simulink library "Feeder1_lib"  (Simulink 8.1)
settings: Solver=ode45  StartTime=0.0  StopTime=10.0  RelTol=1e-3
values from neighbouring files (symbols this model uses):
  DER_REL = xlsread('DER_relay.xlsx')    [relay_settings_init.m]
  Ts = 100E-6    (= 0.0001)    [BANSHEE_init.m]    (also in Ghost_init.m)
undefined symbols (not defined in the file or in its folder): CBID, Left, type, V
libraries: breaker_lib x16, powerlib x11, cables_lib x11, transformer_lib x7, Load_lib x6, ssn_lib x6, NREL_Diesel_Genset_lib x2, rtlab x2, relay_modbus_lib x1, powerlib_meascontrol x1, rtio_generic_modbus x1, Motor_InductionMachine_lib x1
settings Model: Creator=re25624  LastModifiedBy=hptb1

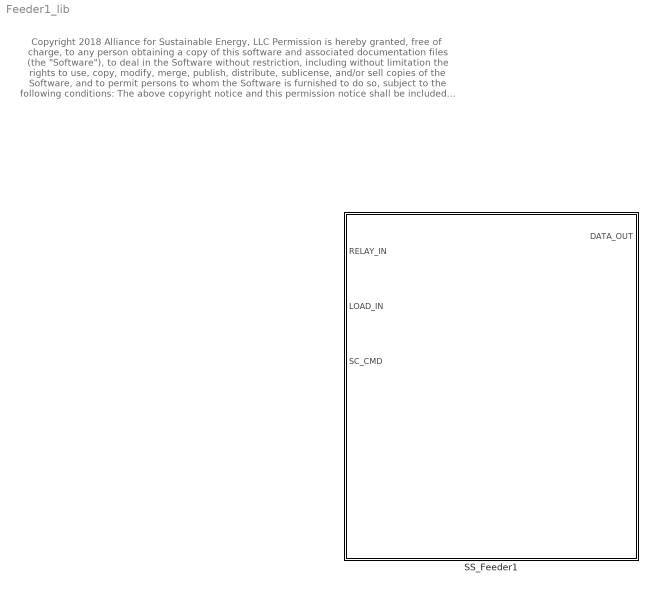
== system Feeder1_lib ==
  note: Copyright 2018 Alliance for Sustainable Energy, LLC
      |
      | Permission is hereby granted, free of charge, to any person obtaining a copy of this software
      | and associated documentation files (the "Software"), to deal in the Software without restriction,
      | including without limitation the rights to use, copy, modify, merge, publish, distribute, sublicense,
      | and/or sell copies of the Software, and to permit persons to whom the Software is furnished to do so,
      | subject to the following conditions:
      |
      | The above copyright notice and this permission notice shall be included in all copies or substantial portions of the Software.
      |
      | THE SOFTWARE IS PROVIDED "AS IS", WITHOUT WARRANTY OF ANY KIND, EXPRESS OR IMPLIED, INCLUDING
      | BUT NOT LIMITED TO THE WARRANTIES OF MERCHANTABILITY, FITNESS FOR A PARTICULAR PURPOSE AND
      | NONINFRINGEMENT. IN NO EVENT SHALL THE AUTHORS, THE COPYRIGHT HOLDERS, THE UNITED STATES,
      | THE UNITED STATES DEPARTMENT OF ENERGY, OR ANY OF THEIR EMPLOYEES BE LIABLE FOR ANY CLAIM,
      | DAMAGES OR OTHER LIABILITY, WHETHER IN AN ACTION OF CONTRACT, TORT OR OTHERWISE, ARISING FROM,
      | OUT OF OR IN CONNECTION WITH THE SOFTWARE OR THE USE OR OTHER DEALINGS IN THE SOFTWARE.
  SS_Feeder1 : Subsystem

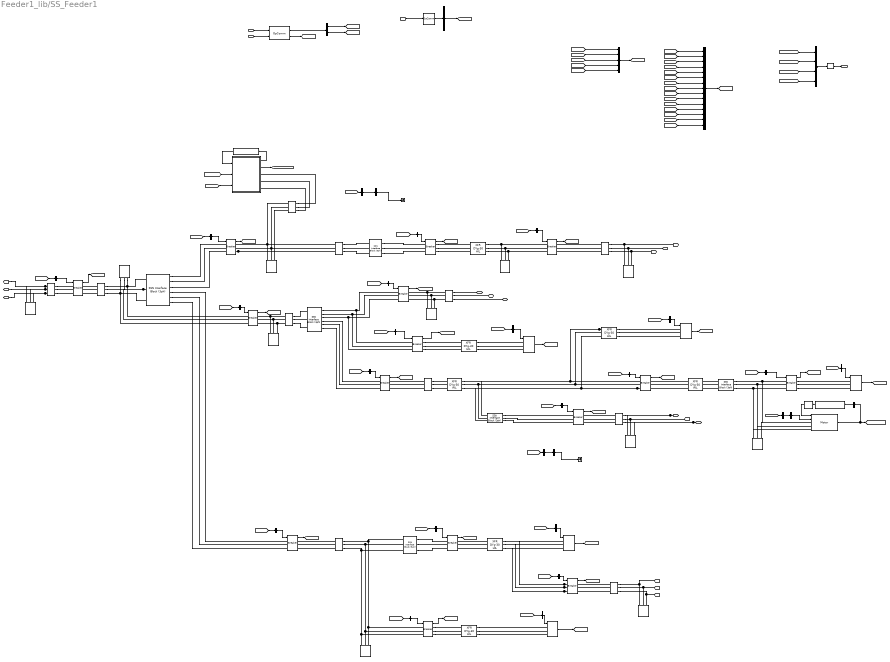
== system Feeder1_lib/SS_Feeder1 ==
  note: Copyright 2018 Alliance for Sustainable Energy, LLC
      |
      | Permission is hereby granted, free of charge, to any person obtaining a copy of this software
      | and associated documentation files (the "Software"), to deal in the Software without restriction,
      | including without limitation the rights to use, copy, modify, merge, publish, distribute, sublicense,
      | and/or sell copies of the Software, and to permit persons to whom the Software is furnished to do so,
      | subject to the following conditions:
      |
      | The above copyright notice and this permission notice shall be included in all copies or substantial portions of the Software.
      |
      | THE SOFTWARE IS PROVIDED "AS IS", WITHOUT WARRANTY OF ANY KIND, EXPRESS OR IMPLIED, INCLUDING
      | BUT NOT LIMITED TO THE WARRANTIES OF MERCHANTABILITY, FITNESS FOR A PARTICULAR PURPOSE AND
      | NONINFRINGEMENT. IN NO EVENT SHALL THE AUTHORS, THE COPYRIGHT HOLDERS, THE UNITED STATES,
      | THE UNITED STATES DEPARTMENT OF ENERGY, OR ANY OF THEIR EMPLOYEES BE LIABLE FOR ANY CLAIM,
      | DAMAGES OR OTHER LIABILITY, WHETHER IN AN ACTION OF CONTRACT, TORT OR OTHERWISE, ARISING FROM,
      | OUT OF OR IN CONNECTION WITH THE SOFTWARE OR THE USE OR OTHER DEALINGS IN THE SOFTWARE.
  note: Copyright 2018 Alliance for Sustainable Energy, LLC
      |
      | Permission is hereby granted, free of charge, to any person obtaining a copy of this software
      | and associated documentation files (the "Software"), to deal in the Software without restriction,
      | including without limitation the rights to use, copy, modify, merge, publish, distribute, sublicense,
      | and/or sell copies of the Software, and to permit persons to whom the Software is furnished to do so,
      | subject to the following conditions:
      |
      | The above copyright notice and this permission notice shall be included in all copies or substantial portions of the Software.
      |
      | THE SOFTWARE IS PROVIDED "AS IS", WITHOUT WARRANTY OF ANY KIND, EXPRESS OR IMPLIED, INCLUDING
      | BUT NOT LIMITED TO THE WARRANTIES OF MERCHANTABILITY, FITNESS FOR A PARTICULAR PURPOSE AND
      | NONINFRINGEMENT. IN NO EVENT SHALL THE AUTHORS, THE COPYRIGHT HOLDERS, THE UNITED STATES,
      | THE UNITED STATES DEPARTMENT OF ENERGY, OR ANY OF THEIR EMPLOYEES BE LIABLE FOR ANY CLAIM,
      | DAMAGES OR OTHER LIABILITY, WHETHER IN AN ACTION OF CONTRACT, TORT OR OTHERWISE, ARISING FROM,
      | OUT OF OR IN CONNECTION WITH THE SOFTWARE OR THE USE OR OTHER DEALINGS IN THE SOFTWARE.
  note: Fault3:
      | Fault Resistance: 0.01Ohm
      | Ground Resistance: 1.73Ohm
      | Snubber resistance: 1E6:
  note: 124kVA to cancel capcitive VARs
      | from stubline
  note: connect to F3
  note: connect to F2
  note: connect to F2
  note: connect to F2
  note: 69kVA to cancel capcitive VARs
      | from stubline
  note: Fault2:
      | Fault Resistance: 0.1Ohm
      | Ground Resistance: 1.73Ohm
      | Snubber resistance: 1E6:
  RELAY_IN : Inport
  LOAD_IN : Inport  Port=2
  SC_CMD : Inport  Port=3
  200 HP chiller compressor : Load_lib/200 HP chiller compressor
  2000 kVA4 : transformer_lib/XFR DYg-30 HIL  Rating=2000  Vp=4160  Vs=480  Z=5.75  XR=5.7
  2000 kVA5 : transformer_lib/XFR DYg-30 HIL  Rating=2000  Vp=4160  Vs=480  Z=5.75  XR=5.7
  2500 kVA : transformer_lib/XFR DYg-30 HIL  Rating=2500  Vp=13800  Vs=480  Z=5.75  XR=6.6
  2500 kVA2 : transformer_lib/XFR DYg-30 HIL  Rating=2500  Vp=13800  Vs=480  Z=5.56  XR=5.52
  3750 kVA1 : transformer_lib/XFR DYg-30 HIL  Rating=3750  Vp=13800  Vs=4160  Z=4.75  XR=11.4
  448 kvar inductor at 13.8kV  to cancel kvar produced by the stublines1 : powerlib/Elements/Three-Phase Parallel RLC Load  LConnTagsString=A|B|C  Configuration=Y (grounded)  NominalVoltage=13800  NominalFrequency=60  ActivePower=10e3  InductivePower=448e3  CapacitivePower=0  Measurements=None  LoadType=constant Z
  5 kvar inductor at 480V  to cancel kvar produced by the stublines : powerlib/Elements/Three-Phase Parallel RLC Load  LConnTagsString=A|B|C  Configuration=Y (grounded)  NominalVoltage=480  NominalFrequency=60  ActivePower=1e3  InductivePower=5e3  CapacitivePower=0  Measurements=None  LoadType=constant Z
  500 kVA2 : transformer_lib/XFR DYg-30 HIL  Rating=500  Vp=13800  Vs=480  Z=5  XR=4.9
  500 kVA3 : transformer_lib/XFR DYg-30 HIL  Rating=500  Vp=13800  Vs=208  Z=5  XR=4.9
  500kcmil-Mutual1 : cables_lib/500kcmil-Mutual  length=1000  par_sets=1  ratio=3
  500kcmil-Mutual9 : cables_lib/500kcmil-Mutual  length=100  par_sets=1  ratio=3
  9 kvar inductor at 480V  to cancel kvar produced by the stublines2 : powerlib/Elements/Three-Phase Parallel RLC Load  LConnTagsString=A|B|C  Configuration=Y (grounded)  NominalVoltage=480  NominalFrequency=60  ActivePower=1e3  InductivePower=9e3  CapacitivePower=0  Measurements=None  LoadType=constant Z
  Bus Creator2 : BusCreator
  Bus Creator3 : BusCreator  Inputs=5
  Bus Creator5 : BusCreator  Inputs=15
  Bus Selector : BusSelector  OutputSignals=motor
  Bus Selector1 : BusSelector  OutputSignals=F1_CB_12
  Bus Selector10 : BusSelector  OutputSignals=F1_CB_2
  Bus Selector11 : BusSelector  OutputSignals=F1_CB_1
  Bus Selector12 : BusSelector  OutputSignals=F1_CB_5
  Bus Selector13 : BusSelector  OutputSignals=F1_CB_3
  Bus Selector14 : BusSelector  OutputSignals=F1_CB_6
  Bus Selector15 : BusSelector  OutputSignals=F1_CB_7
  Bus Selector16 : BusSelector  OutputSignals=F1_CB_10
  Bus Selector17 : BusSelector  OutputSignals=F1_CB_11
  Bus Selector18 : BusSelector  OutputSignals=F1_CB_9
  Bus Selector19 : BusSelector  OutputSignals=F1_CB_14
  Bus Selector2 : BusSelector  OutputSignals=F1_CB_4
  Bus Selector20 : BusSelector  OutputSignals=Gen1
  Bus Selector21 : BusSelector  OutputSignals=LoadProfile,TestSeq
  Bus Selector22 : BusSelector  OutputSignals=RPM
  Bus Selector23 : BusSelector  OutputSignals=ena1
  Bus Selector24 : BusSelector  OutputSignals=fault
  Bus Selector25 : BusSelector  OutputSignals=loc2
  Bus Selector26 : BusSelector  OutputSignals=F1_PCC
  Bus Selector27 : BusSelector  OutputSignals=fault
  Bus Selector28 : BusSelector  OutputSignals=loc3
  Bus Selector3 : BusSelector  OutputSignals=I2
  Bus Selector4 : BusSelector  OutputSignals=C2
  Bus Selector5 : BusSelector  OutputSignals=P1
  Bus Selector6 : BusSelector  OutputSignals=C1
  Bus Selector7 : BusSelector  OutputSignals=I1
  Bus Selector8 : BusSelector  OutputSignals=F1_CB_13
  Bus Selector9 : BusSelector  OutputSignals=F1_CB_8
  C{1..2,108..109} (4 alike) : cables_lib/500kcmil-Mutual  length=10  par_sets=1  ratio=3
  C101 : cables_lib/500kcmil-Mutual  length=1800  par_sets=1  ratio=3
  C102 : cables_lib/500kcmil-Mutual  length=5500  par_sets=1  ratio=3
  C103 : cables_lib/4//0AWG-Mutual  length=1000  par_sets=1  ratio=3
  C104 : cables_lib/500kcmil-Mutual  length=3000  par_sets=1  ratio=3
  C106 : cables_lib/500kcmil-Mutual  length=1500  par_sets=1  ratio=3
  Critical_1 : Load_lib/Dynamic_Load  V=480  kVA=1200  PF=0.9  Ts=Ts
  Critical_2 : Load_lib/Dynamic_Load  V=480  kVA=1500  PF=0.9  Ts=Ts
  Diesel_Generator1 : Subsystem
  F1_CB_{1..14} (14 alike) : breaker_lib/Breaker  Ts=Ts  mech_delay=cb_mech_delay
  F1_PCC : breaker_lib/Breaker  Ts=Ts  mech_delay=cb_mech_delay
  First-Order Filter : powerlib_meascontrol/Filters/First-Order Filter  FilterType=Lowpass  Tc=10e-3  Ts=Ts  Initialize=on  Vac_Init=[0, 0, 60]  Vdc_Init=0  PlotResponse=off  FreqRange="[0,  200,  1]"
  GEN3_Modbus : rtio_generic_modbus/Modbus device  conf_name=GEN1_modbus.opal  conf_name_mask=GEN1_modbus.xls  sample_time=Ts
  Interruptible_1 : Load_lib/Dynamic_Load  V=480  kVA=300  PF=0.9  Ts=Ts
  Interruptible_2 : Load_lib/Dynamic_Load  V=208  kVA=250  PF=0.9  Ts=Ts
  Losses{1..2,4,6} (4 alike) : powerlib/Elements/Three-Phase Parallel RLC Load  LConnTagsString=A|B|C  Configuration=Y (grounded)  NominalVoltage=13800  NominalFrequency=60  ActivePower=1e3  InductivePower=0  CapacitivePower=0  Measurements=None  LoadType=constant Z
  Losses3 : powerlib/Elements/Three-Phase Parallel RLC Load  LConnTagsString=A|B|C  Configuration=Y (grounded)  NominalVoltage=480  NominalFrequency=60  ActivePower=1e3  InductivePower=0  CapacitivePower=0  Measurements=None  LoadType=constant Z
  Losses5 : powerlib/Elements/Three-Phase Parallel RLC Load  LConnTagsString=A|B|C  Configuration=Y (grounded)  NominalVoltage=480  NominalFrequency=60  ActivePower=1e3  InductivePower=0  CapacitivePower=0  Measurements=None  LoadType=constant Z
  Losses7 : powerlib/Elements/Three-Phase Parallel RLC Load  LConnTagsString=A|B|C  Configuration=Y (grounded)  NominalVoltage=13800  NominalFrequency=60  ActivePower=1e3  InductivePower=124e3  CapacitivePower=0  Measurements=None  LoadType=constant Z
  Losses8 : powerlib/Elements/Three-Phase Parallel RLC Load  LConnTagsString=A|B|C  Configuration=Y (grounded)  NominalVoltage=4160  NominalFrequency=60  ActivePower=1e3  InductivePower=69e3  CapacitivePower=0  Measurements=None  LoadType=constant Z
  Memory : Memory
  Motor : Motor_InductionMachine_lib/Motor
  OpComm1 : rtlab/OpComm  nbport=2  groupe_acq=1  subsys_rate=0  st=0  Synchronization=on  Interpolation=on  Threshold=1.0  Missed_Data=off  Sim_Time=off  Samples=off  dynSigOut=off  from_console=0  warning_done=off  writeOpCommFile=off  Offset=off
  OpComm2 : rtlab/OpComm  nbport=1  groupe_acq=1  subsys_rate=0  st=0  Synchronization=on  Interpolation=on  Threshold=1.0  Missed_Data=off  Sim_Time=off  Samples=off  dynSigOut=off  from_console=1  warning_done=off  writeOpCommFile=off  Offset=off
  Priority_1 : Load_lib/Dynamic_Load  V=480  kVA=1000  PF=0.9  Ts=Ts
  SSN Interface Block (3ph) : ssn_lib/SSN Interface Block (3ph)  nb_phase=3  nb_port=3  p1_type=V-type(Left)  p2_type=V-type (Right)  p3_type=V-type (Right)  p4_type=V-type (Right)  p5_type=V-type(Left)  p6_type=V-type(Left)  p7_type=V-type(Left)  p8_type=V-type(Left)  p9_type=V-type(Left)  p10_type=V-type(Left)  p11_type=V-type(Left)  p12_type=V-type(Left)  p13_type=V-type(Left)  p14_type=V-type(Left)  p15_type=V-type(Left)  p16_type=V-type(Left)  I_port_shunt_resistance=1e9
  SSN Interface Block (3ph)1 : ssn_lib/SSN Interface Block (3ph)  nb_phase=3  nb_port=3  p1_type=V-type(Left)  p2_type=V-type (Right)  p3_type=V-type (Right)  p4_type=V-type(Left)  p5_type=V-type(Left)  p6_type=V-type(Left)  p7_type=V-type(Left)  p8_type=V-type(Left)  p9_type=V-type(Left)  p10_type=V-type(Left)  p11_type=V-type(Left)  p12_type=V-type(Left)  p13_type=V-type(Left)  p14_type=V-type(Left)  p15_type=V-type(Left)  p16_type=V-type(Left)  I_port_shunt_resistance=1e9
  SSN Interface Block (3ph){2..4,12} (4 alike) : ssn_lib/SSN Interface Block (3ph)  nb_phase=3  nb_port=2  p1_type=V-type(Left)  p2_type=V-type (Right)  p3_type=V-type(Left)  p4_type=V-type(Left)  p5_type=V-type(Left)  p6_type=V-type(Left)  p7_type=V-type(Left)  p8_type=V-type(Left)  p9_type=V-type(Left)  p10_type=V-type(Left)  p11_type=V-type(Left)  p12_type=V-type(Left)  p13_type=V-type(Left)  p14_type=V-type(Left)  p15_type=V-type(Left)  p16_type=V-type(Left)  I_port_shunt_resistance=1e9
  Terminator : Terminator
  Terminator1 : Terminator
  A_CB_8 : PMIOPort  Port=1  Side=Right
  B_CB_8 : PMIOPort  Port=2  Side=Right
  C_CB_8 : PMIOPort  Port=3  Side=Right
  A_CB_11 : PMIOPort  Port=4  Side=Right
  B_CB_11 : PMIOPort  Port=5  Side=Right
  C_CB_11 : PMIOPort  Port=6  Side=Right
  A_CB_9 : PMIOPort  Port=7  Side=Right
  B_CB_9 : PMIOPort  Port=8  Side=Right
  C_CB_9 : PMIOPort  Port=9  Side=Right
  A_CB_13 : PMIOPort  Port=10  Side=Right
  B_CB_13 : PMIOPort  Port=11  Side=Right
  C_CB_13 : PMIOPort  Port=12  Side=Right
  PCC_A : PMIOPort  Port=13  Side=Left
  PCC_B : PMIOPort  Port=14  Side=Left
  PCC_C : PMIOPort  Port=15  Side=Left
  DATA_OUT : Outport
  wires:
  Bus Selector28/1 -> Terminator1/1  "<loc3>"
  Bus Selector27/1 -> Bus Selector28/1  "<fault>"
  [TestSeq] -> Bus Selector27/1
  Bus Selector25/1 -> Terminator/1  "<loc2>"
  Bus Selector24/1 -> Bus Selector25/1  "<fault>"
  [TestSeq] -> Bus Selector24/1
  First-Order Filter/1 -> Motor/1
  [TestSeq] -> Diesel_Generator1/3(testseq)
  [MOTOR_DATA] -> Bus Creator2/4  "MOTOR_DATA"
  Bus Selector23/1 -> Motor/2  "<ena1>"
  Bus Selector21/2 -> [TestSeq]  "<TestSeq>"
  Bus Selector21/1 -> [LOAD_IN]  "<LoadProfile>"
  OpComm1/1 -> Bus Selector21/1
  Diesel_Generator1/2(Gen_meas) -> [DIESEL_DATA]
  Diesel_Generator1/1(ModbusOut) -> GEN3_Modbus/1  "Gen_meas"
  GEN3_Modbus/1 -> Diesel_Generator1/1(ModbusIn)
  [Gen1] -> Diesel_Generator1/2(console)
  [RELAY_IN] -> Bus Selector26/1
  Bus Selector26/1 -> F1_PCC/1  "<F1_PCC>"
  Bus Selector/1 -> Bus Selector23/1  "<motor>"
  [TestSeq] -> Bus Selector/1
  Bus Selector20/1 -> [Gen1]  "<Gen1>"
  200 HP chiller compressor/1 -> First-Order Filter/1
  Bus Selector22/1 -> 200 HP chiller compressor/1  "<RPM>"
  Motor/1 -> Bus Selector22/1, [MOTOR_DATA]
  [DIESEL_DATA] -> Bus Creator2/3  "DIESEL_DATA"
  [LOAD_DATA] -> Bus Creator2/2  "LOAD_DATA"
  [CB_DATA] -> Bus Creator2/1  "CB_DATA"
  Bus Creator2/1 -> Memory/1
  Memory/1 -> DATA_OUT/1
  Bus Creator5/1 -> [CB_DATA]
  Bus Creator3/1 -> [LOAD_DATA]  "LOAD"
  OpComm2/1 -> Bus Selector20/1
  SC_CMD/1 -> OpComm2/1
  [F1_CB_14] -> Bus Creator5/14  "F1_CB_14"
  [F1_PCC] -> Bus Creator5/15  "F1_PCC"
  Bus Selector19/1 -> F1_CB_14/1  "<F1_CB_14>"
  [RELAY_IN] -> Bus Selector19/1
  F1_CB_14/1 -> [F1_CB_14]
  Bus Selector2/1 -> F1_CB_4/1  "<F1_CB_4>"
  [RELAY_IN] -> Bus Selector2/1
  F1_CB_4/1 -> [F1_CB_4]
  F1_CB_2/1 -> [F1_CB_2]
  Bus Selector18/1 -> F1_CB_9/1  "<F1_CB_9>"
  Bus Selector12/1 -> F1_CB_5/1  "<F1_CB_5>"
  Bus Selector11/1 -> F1_CB_1/1  "<F1_CB_1>"
  Bus Selector17/1 -> F1_CB_11/1  "<F1_CB_11>"
  Bus Selector16/1 -> F1_CB_10/1  "<F1_CB_10>"
  Bus Selector10/1 -> F1_CB_2/1  "<F1_CB_2>"
  Bus Selector14/1 -> F1_CB_6/1  "<F1_CB_6>"
  Bus Selector15/1 -> F1_CB_7/1  "<F1_CB_7>"
  Bus Selector9/1 -> F1_CB_8/1  "<F1_CB_8>"
  Bus Selector8/1 -> F1_CB_13/1  "<F1_CB_13>"
  Bus Selector1/1 -> F1_CB_12/1  "<F1_CB_12>"
  [RELAY_IN] -> Bus Selector18/1
  [RELAY_IN] -> Bus Selector17/1
  [RELAY_IN] -> Bus Selector16/1
  [RELAY_IN] -> Bus Selector15/1
  [RELAY_IN] -> Bus Selector14/1
  [RELAY_IN] -> Bus Selector12/1
  [RELAY_IN] -> Bus Selector11/1
  [RELAY_IN] -> Bus Selector10/1
  [RELAY_IN] -> Bus Selector9/1
  [RELAY_IN] -> Bus Selector8/1
  [RELAY_IN] -> Bus Selector1/1
  [RELAY_IN] -> Bus Selector13/1
  Bus Selector13/1 -> F1_CB_3/1  "<F1_CB_3>"
  OpComm1/2 -> [RELAY_IN]
  RELAY_IN/1 -> OpComm1/2
  [F1_CB_2] -> Bus Creator5/2  "F1_CB_2"
  [F1_CB_3] -> Bus Creator5/3  "F1_CB_3"
  [F1_CB_4] -> Bus Creator5/4  "F1_CB_4"
  [F1_CB_5] -> Bus Creator5/5  "F1_CB_5"
  [F1_CB_6] -> Bus Creator5/6  "F1_CB_6"
  [F1_CB_7] -> Bus Creator5/7  "F1_CB_7"
  [F1_CB_8] -> Bus Creator5/8  "F1_CB_8"
  [F1_CB_9] -> Bus Creator5/9  "F1_CB_9"
  [F1_CB_10] -> Bus Creator5/10  "F1_CB_10"
  [F1_CB_11] -> Bus Creator5/11  "F1_CB_11"
  [F1_CB_12] -> Bus Creator5/12  "F1_CB_12"
  [F1_CB_13] -> Bus Creator5/13  "F1_CB_13"
  [F1_CB_1] -> Bus Creator5/1  "F1_CB_1"
  F1_CB_11/1 -> [F1_CB_11]
  F1_CB_10/1 -> [F1_CB_10]
  F1_CB_13/1 -> [F1_CB_13]
  F1_CB_12/1 -> [F1_CB_12]
  F1_CB_8/1 -> [F1_CB_8]
  F1_CB_7/1 -> [F1_CB_7]
  F1_CB_6/1 -> [F1_CB_6]
  F1_CB_9/1 -> [F1_CB_9]
  F1_CB_5/1 -> [F1_CB_5]
  F1_CB_1/1 -> [F1_CB_1]
  F1_CB_3/1 -> [F1_CB_3]
  [LOAD_I1] -> Bus Creator3/3  "F1_I1"
  [LOAD_C2] -> Bus Creator3/2  "F1_C2"
  [LOAD_P1] -> Bus Creator3/5  "F1_P1"
  [LOAD_I2] -> Bus Creator3/4  "F1_I2"
  [LOAD_C1] -> Bus Creator3/1  "F1_C1"
  Interruptible_1/1 -> [LOAD_I1]
  Critical_1/1 -> [LOAD_C1]
  Priority_1/1 -> [LOAD_P1]
  Critical_2/1 -> [LOAD_C2]
  Interruptible_2/1 -> [LOAD_I2]
  Bus Selector7/1 -> Interruptible_1/1  "<I1>"
  Bus Selector6/1 -> Critical_1/1  "<C1>"
  Bus Selector5/1 -> Priority_1/1  "<P1>"
  Bus Selector4/1 -> Critical_2/1  "<C2>"
  Bus Selector3/1 -> Interruptible_2/1  "<I2>"
  [LOAD_IN] -> Bus Selector7/1
  [LOAD_IN] -> Bus Selector6/1
  [LOAD_IN] -> Bus Selector5/1
  [LOAD_IN] -> Bus Selector4/1
  [LOAD_IN] -> Bus Selector3/1
  LOAD_IN/1 -> OpComm1/1
  F1_PCC/1 -> [F1_PCC]
  connections:
  C103/RConn1 -- Diesel_Generator1/RConn1
  C103/RConn2 -- Diesel_Generator1/RConn2
  Losses7/LConn2 -- C2/LConn2 -- F1_CB_8/RConn2
  Losses7/LConn1 -- F1_CB_8/RConn1 -- C2/LConn1
  Losses7/LConn3 -- C2/LConn3 -- F1_CB_8/RConn3
  C1/LConn1 -- F1_CB_11/RConn1
  C1/LConn2 -- F1_CB_11/RConn2
  C1/LConn3 -- F1_CB_11/RConn3
  C_CB_11/RConn1 -- Losses8/LConn3 -- C1/RConn3
  A_CB_11/RConn1 -- Losses8/LConn1 -- C1/RConn1
  B_CB_11/RConn1 -- C1/RConn2 -- Losses8/LConn2
  C2/RConn3 -- C_CB_8/RConn1
  C2/RConn2 -- B_CB_8/RConn1
  C2/RConn1 -- A_CB_8/RConn1
  500kcmil-Mutual1/LConn1 -- 448 kvar inductor at 13.8kV  to cancel kvar produced by the stublines1/LConn1 -- PCC_A/RConn1
  500kcmil-Mutual1/LConn3 -- 448 kvar inductor at 13.8kV  to cancel kvar produced by the stublines1/LConn3 -- PCC_C/RConn1
  500kcmil-Mutual1/LConn2 -- 448 kvar inductor at 13.8kV  to cancel kvar produced by the stublines1/LConn2 -- PCC_B/RConn1
  500kcmil-Mutual9/RConn1 -- Losses1/LConn3 -- F1_CB_2/LConn1 -- SSN Interface Block (3ph)/LConn1
  Losses1/LConn1 -- SSN Interface Block (3ph)/LConn3 -- F1_CB_2/LConn3 -- 500kcmil-Mutual9/RConn3
  SSN Interface Block (3ph)/LConn2 -- Losses1/LConn2 -- F1_CB_2/LConn2 -- 500kcmil-Mutual9/RConn2
  500kcmil-Mutual1/RConn1 -- F1_PCC/LConn1
  500kcmil-Mutual1/RConn2 -- F1_PCC/LConn2
  500kcmil-Mutual1/RConn3 -- F1_PCC/LConn3
  500kcmil-Mutual9/LConn3 -- F1_PCC/RConn3
  500kcmil-Mutual9/LConn1 -- F1_PCC/RConn1
  500kcmil-Mutual9/LConn2 -- F1_PCC/RConn2
  9 kvar inductor at 480V  to cancel kvar produced by the stublines2/LConn3 -- C108/RConn3 -- C_CB_9/RConn1
  9 kvar inductor at 480V  to cancel kvar produced by the stublines2/LConn1 -- C108/RConn1 -- A_CB_9/RConn1
  9 kvar inductor at 480V  to cancel kvar produced by the stublines2/LConn2 -- C108/RConn2 -- B_CB_9/RConn1
  5 kvar inductor at 480V  to cancel kvar produced by the stublines/LConn1 -- C109/RConn1 -- A_CB_13/RConn1
  5 kvar inductor at 480V  to cancel kvar produced by the stublines/LConn2 -- C109/RConn2 -- B_CB_13/RConn1
  5 kvar inductor at 480V  to cancel kvar produced by the stublines/LConn3 -- C109/RConn3 -- C_CB_13/RConn1
  500 kVA2/RConn1 -- Interruptible_1/LConn1
  500 kVA2/RConn2 -- Interruptible_1/LConn2
  500 kVA2/RConn3 -- Interruptible_1/LConn3
  SSN Interface Block (3ph)4/LConn1 -- 2000 kVA5/RConn1
  SSN Interface Block (3ph)4/LConn2 -- 2000 kVA5/RConn2
  SSN Interface Block (3ph)4/LConn3 -- 2000 kVA5/RConn3
  2000 kVA4/RConn2 -- Critical_2/LConn2
  2000 kVA4/RConn1 -- Critical_2/LConn1
  2000 kVA4/RConn3 -- Critical_2/LConn3
  500 kVA3/RConn1 -- Interruptible_2/LConn1
  500 kVA3/RConn2 -- Interruptible_2/LConn2
  500 kVA3/RConn3 -- Interruptible_2/LConn3
  C103/RConn3 -- Diesel_Generator1/RConn3
  F1_CB_14/LConn1 -- SSN Interface Block (3ph)4/RConn1 -- Losses5/LConn3 -- Motor/LConn1
  F1_CB_14/LConn3 -- SSN Interface Block (3ph)4/RConn3 -- Losses5/LConn1 -- Motor/LConn3
  F1_CB_14/LConn2 -- SSN Interface Block (3ph)4/RConn2 -- Losses5/LConn2 -- Motor/LConn2
  C106/RConn1 -- 3750 kVA1/LConn1
  C106/RConn3 -- 3750 kVA1/LConn3
  C106/RConn2 -- 3750 kVA1/LConn2
  SSN Interface Block (3ph)1/RConn5 -- F1_CB_6/LConn2
  SSN Interface Block (3ph)1/RConn4 -- F1_CB_6/LConn1
  SSN Interface Block (3ph)1/RConn6 -- F1_CB_6/LConn3
  F1_CB_7/LConn3 -- SSN Interface Block (3ph)1/RConn3 -- F1_CB_8/LConn3
  F1_CB_7/LConn2 -- SSN Interface Block (3ph)1/RConn2 -- F1_CB_8/LConn2
  F1_CB_7/LConn1 -- SSN Interface Block (3ph)1/RConn1 -- F1_CB_8/LConn1
  2000 kVA4/LConn1 -- 3750 kVA1/RConn1 -- SSN Interface Block (3ph)12/LConn1 -- F1_CB_10/LConn1
  SSN Interface Block (3ph)12/RConn2 -- F1_CB_11/LConn2
  F1_CB_10/LConn3 -- 3750 kVA1/RConn3 -- SSN Interface Block (3ph)12/LConn3 -- 2000 kVA4/LConn3
  SSN Interface Block (3ph)3/RConn3 -- F1_CB_12/LConn3
  SSN Interface Block (3ph)3/RConn1 -- F1_CB_12/LConn1
  SSN Interface Block (3ph)3/RConn2 -- F1_CB_12/LConn2
  C104/RConn1 -- SSN Interface Block (3ph)3/LConn1
  C104/RConn3 -- SSN Interface Block (3ph)3/LConn3
  C104/RConn2 -- SSN Interface Block (3ph)3/LConn2
  C109/LConn2 -- F1_CB_13/RConn2
  C109/LConn3 -- F1_CB_13/RConn3
  C109/LConn1 -- F1_CB_13/RConn1
  SSN Interface Block (3ph)/RConn3 -- F1_CB_3/LConn3
  SSN Interface Block (3ph)/RConn2 -- F1_CB_3/LConn2
  SSN Interface Block (3ph)/RConn1 -- F1_CB_3/LConn1
  SSN Interface Block (3ph)2/RConn3 -- F1_CB_5/LConn3
  SSN Interface Block (3ph)2/RConn1 -- F1_CB_5/LConn1
  SSN Interface Block (3ph)2/RConn2 -- F1_CB_5/LConn2
  F1_CB_14/RConn3 -- Priority_1/LConn3
  F1_CB_14/RConn2 -- Priority_1/LConn2
  F1_CB_14/RConn1 -- Priority_1/LConn1
  F1_CB_4/RConn2 -- 500 kVA2/LConn2
  F1_CB_4/RConn3 -- 500 kVA2/LConn3
  F1_CB_4/RConn1 -- 500 kVA2/LConn1
  SSN Interface Block (3ph)12/RConn1 -- F1_CB_11/LConn1
  3750 kVA1/RConn2 -- SSN Interface Block (3ph)12/LConn2 -- F1_CB_10/LConn2 -- 2000 kVA4/LConn2
  SSN Interface Block (3ph)12/RConn3 -- F1_CB_11/LConn3
  F1_CB_9/LConn3 -- Critical_1/LConn3 -- 2500 kVA2/RConn3
  F1_CB_4/LConn1 -- Losses6/LConn3 -- SSN Interface Block (3ph)2/LConn1 -- C101/RConn1
  Losses3/LConn3 -- 2500 kVA/RConn3 -- F1_CB_13/LConn3
  F1_CB_4/LConn2 -- Losses6/LConn2 -- SSN Interface Block (3ph)2/LConn2 -- C101/RConn2
  F1_CB_7/RConn2 -- 500 kVA3/LConn2
  F1_CB_7/RConn1 -- 500 kVA3/LConn1
  Losses3/LConn1 -- 2500 kVA/RConn1 -- F1_CB_13/LConn1
  C108/LConn3 -- F1_CB_9/RConn3
  F1_CB_3/RConn3 -- Losses2/LConn3 -- C103/LConn3 -- C104/LConn3
  C101/LConn3 -- F1_CB_1/RConn3
  C108/LConn2 -- F1_CB_9/RConn2
  C108/LConn1 -- F1_CB_9/RConn1
  Losses2/LConn1 -- F1_CB_3/RConn1 -- C103/LConn1 -- C104/LConn1
  2000 kVA5/LConn3 -- F1_CB_10/RConn3
  C101/LConn2 -- F1_CB_1/RConn2
  F1_CB_7/RConn3 -- 500 kVA3/LConn3
  F1_CB_12/RConn3 -- 2500 kVA/LConn3
  C101/LConn1 -- F1_CB_1/RConn1
  F1_CB_12/RConn2 -- 2500 kVA/LConn2
  2000 kVA5/LConn2 -- F1_CB_10/RConn2
  C106/LConn3 -- F1_CB_6/RConn3
  Losses2/LConn2 -- F1_CB_3/RConn2 -- C103/LConn2 -- C104/LConn2
  2500 kVA2/LConn1 -- F1_CB_5/RConn1
  2000 kVA5/LConn1 -- F1_CB_10/RConn1
  C106/LConn2 -- F1_CB_6/RConn2
  SSN Interface Block (3ph)/RConn4 -- F1_CB_1/LConn1
  SSN Interface Block (3ph)/RConn5 -- F1_CB_1/LConn2
  SSN Interface Block (3ph)/RConn6 -- F1_CB_1/LConn3
  F1_CB_12/RConn1 -- 2500 kVA/LConn1
  F1_CB_4/LConn3 -- Losses6/LConn1 -- SSN Interface Block (3ph)2/LConn3 -- C101/RConn3
  F1_CB_9/LConn1 -- Critical_1/LConn1 -- 2500 kVA2/RConn1
  Losses4/LConn1 -- C102/LConn1 -- F1_CB_2/RConn1
  Losses4/LConn3 -- C102/LConn3 -- F1_CB_2/RConn3
  2500 kVA2/LConn2 -- F1_CB_5/RConn2
  Losses4/LConn2 -- C102/LConn2 -- F1_CB_2/RConn2
  2500 kVA2/LConn3 -- F1_CB_5/RConn3
  Losses3/LConn2 -- 2500 kVA/RConn2 -- F1_CB_13/LConn2
  C106/LConn1 -- F1_CB_6/RConn1
  F1_CB_9/LConn2 -- Critical_1/LConn2 -- 2500 kVA2/RConn2
  C102/RConn2 -- SSN Interface Block (3ph)1/LConn2
  C102/RConn3 -- SSN Interface Block (3ph)1/LConn3
  C102/RConn1 -- SSN Interface Block (3ph)1/LConn1

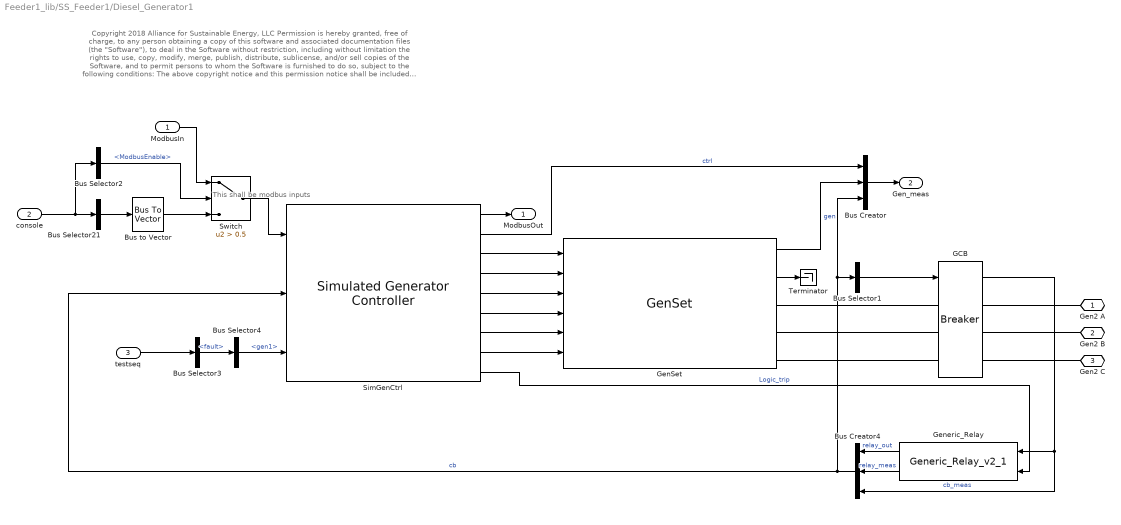
== system Feeder1_lib/SS_Feeder1/Diesel_Generator1 ==
  note: Copyright 2018 Alliance for Sustainable Energy, LLC
      |
      | Permission is hereby granted, free of charge, to any person obtaining a copy of this software
      | and associated documentation files (the "Software"), to deal in the Software without restriction,
      | including without limitation the rights to use, copy, modify, merge, publish, distribute, sublicense,
      | and/or sell copies of the Software, and to permit persons to whom the Software is furnished to do so,
      | subject to the following conditions:
      |
      | The above copyright notice and this permission notice shall be included in all copies or substantial portions of the Software.
      |
      | THE SOFTWARE IS PROVIDED "AS IS", WITHOUT WARRANTY OF ANY KIND, EXPRESS OR IMPLIED, INCLUDING
      | BUT NOT LIMITED TO THE WARRANTIES OF MERCHANTABILITY, FITNESS FOR A PARTICULAR PURPOSE AND
      | NONINFRINGEMENT. IN NO EVENT SHALL THE AUTHORS, THE COPYRIGHT HOLDERS, THE UNITED STATES,
      | THE UNITED STATES DEPARTMENT OF ENERGY, OR ANY OF THEIR EMPLOYEES BE LIABLE FOR ANY CLAIM,
      | DAMAGES OR OTHER LIABILITY, WHETHER IN AN ACTION OF CONTRACT, TORT OR OTHERWISE, ARISING FROM,
      | OUT OF OR IN CONNECTION WITH THE SOFTWARE OR THE USE OR OTHER DEALINGS IN THE SOFTWARE.
  note: This shall be modbus inputs
  ModbusIn : Inport
  console : Inport  Port=2
  testseq : Inport  Port=3
  Bus Creator : BusCreator  Inputs=3
  Bus Creator4 : BusCreator  Inputs=3
  Bus Selector1 : BusSelector  OutputSignals=relay_out  OutputAsBus=on
  Bus Selector2 : BusSelector  OutputSignals=ModbusEnable
  Bus Selector21 : BusSelector  OutputSignals=ModbusFromSC.Ctrl,ModbusFromSC.PCmd,ModbusFromSC.QCmd,ModbusFromSC.VoltCmd,ModbusFromSC.FreqCmd,ModbusFromSC.signal6,ModbusFromSC.signal7,ModbusFromSC.signal8  OutputAsBus=on
  Bus Selector3 : BusSelector  OutputSignals=fault
  Bus Selector4 : BusSelector  OutputSignals=gen1
  Bus to Vector : BusToVector
  GCB : breaker_lib/Breaker  Ts=Ts  mech_delay=cb_mech_delay
  GenSet : NREL_Diesel_Genset_lib/GenSet  GenSel=4MVA diesel generator
  Generic_Relay : relay_modbus_lib/Generic_Relay_v2_1  Ts=Ts  relay_settings=[DER_REL(CBID.GEN1,:)]
  SimGenCtrl : NREL_Diesel_Genset_lib/Simulated Generator Controller  GenSel=4MVA diesel generator
  Switch : Switch  Criteria=u2 > Threshold  Threshold=0.5
  Terminator : Terminator
  Gen2 A : PMIOPort  Port=1  Side=Right
  Gen2 B : PMIOPort  Port=2  Side=Right
  Gen2 C : PMIOPort  Port=3  Side=Right
  ModbusOut : Outport
  Gen_meas : Outport  Port=2
  wires:
  Bus Selector1/1 -> GCB/1
  Bus Selector4/1 -> SimGenCtrl/3  "<gen1>"
  Bus Selector3/1 -> Bus Selector4/1  "<fault>"
  testseq/1 -> Bus Selector3/1
  GenSet/2 -> Terminator/1
  SimGenCtrl/2 -> Bus Creator/1  "ctrl"
  Bus Creator/1 -> Gen_meas/1
  Generic_Relay/2 -> Bus Creator4/2  "relay_meas"
  Generic_Relay/1 -> Bus Creator4/1  "relay_out"
  GCB/1 -> Bus Creator4/3, Generic_Relay/1  "cb_meas"
  Switch/1 -> SimGenCtrl/1
  Bus to Vector/1 -> Switch/3
  Bus Selector21/1 -> Bus to Vector/1
  ModbusIn/1 -> Switch/1
  Bus Selector2/1 -> Switch/2  "<ModbusEnable>"
  console/1 -> Bus Selector2/1, Bus Selector21/1
  Bus Creator4/1 -> SimGenCtrl/2, Bus Selector1/1, Bus Creator/3  "cb"
  GenSet/1 -> Bus Creator/2  "gen"
  SimGenCtrl/6 -> GenSet/4
  SimGenCtrl/5 -> GenSet/3
  SimGenCtrl/4 -> GenSet/2
  SimGenCtrl/3 -> GenSet/1
  SimGenCtrl/7 -> GenSet/5
  SimGenCtrl/8 -> GenSet/6
  SimGenCtrl/1 -> ModbusOut/1
  SimGenCtrl/9 -> Generic_Relay/2  "Logic_trip"
  connections:
  GenSet/RConn3 -- GCB/LConn3
  GenSet/RConn2 -- GCB/LConn2
  GenSet/RConn1 -- GCB/LConn1
  Gen2 C/RConn1 -- GCB/RConn3
  GCB/RConn2 -- Gen2 B/RConn1
  Gen2 A/RConn1 -- GCB/RConn1
